simulink model "smo13"  (R2023a)
settings: Solver=VariableStepAuto  StartTime=0.0  StopTime=100  RelTol=1e-3
model workspace (MAT data in the model file):
  MaxTaskWeight = 2
  lambda = 1
  mu = 1
values from neighbouring files (symbols this model uses):
  m = m + 1    (= 2)    [TMO5liubimov.m]    (also in laba2.m = 14; laba3.m = 200; test.m = 5)
  n = 31    [laba2.m]    (also in test.m = 7)
settings Model: PacingRate=1000  Creator=error  LastModifiedBy=error

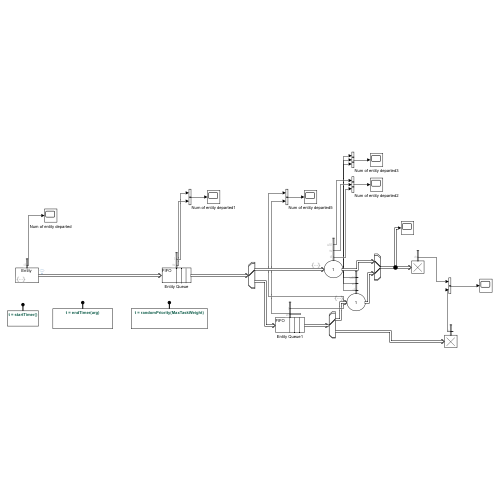
[thumbnail: Simulink's stored preview of the top-level diagram]
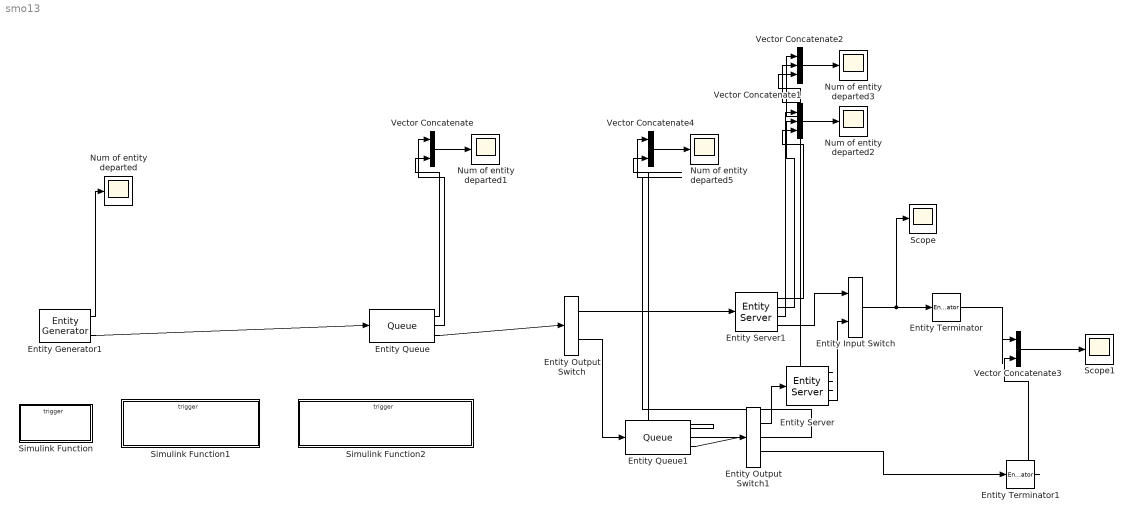
== system smo13 ==
  Entity Input Switch : EntityInputSwitch  InputPortMessageModes=m,m  OutputPortMessageModes=m
  Entity Output Switch : EntityOutputSwitch  InputPortMessageModes=m  OutputPortMessageModes=m,m  SwitchAttributeName=Attribute1
  Entity Output Switch1 : EntityOutputSwitch  InputPortMessageModes=m  OutputPortMessageModes=m,m  SwitchAttributeName=Attribute1
  Entity Generator1 : EntityGenerator  OutputPortMessageModes=n,m  TimeSource=MATLAB action  IntergenerationTimeAction=|  GenerateAction=|  AttributeName=ServiceTime|arrivalTime|time|priority  AttributeInitialValue=exprnd(1/mu);|0|0|0  NumberEntitiesDeparted=on  EntityType=Structured  EntityTypeName=Entity
      IntergenerationTimeAction=|
      | persistent rngInit;
      | if isempty(rngInit)
      |     rng(12345);
      |     rngInit = true;
      | end
      | 
      | dt = exprnd(1/lambda);
      GenerateAction=|
      | entity.arrivalTime = startTimer();
      | entity.priority = randomPriority(MaxTaskWeight+5);
      settings: OutputPortMap=o0,o3
  Entity Queue : Queue  InputPortMessageModes=m  OutputPortMessageModes=n,n,m  AverageWait=on  AverageQueueLength=on
      settings: OutputPortMap=o2,o3,o5
  Entity Queue1 : Queue  InputPortMessageModes=m  OutputPortMessageModes=n,n,m  Capacity=1  PrioritySource=priority  AverageWait=on  AverageQueueLength=on
      settings: OutputPortMap=o2,o3,o5
  Entity Server : EntityServer  InputPortMessageModes=m  OutputPortMessageModes=n,n,n,m  Capacity=1  ServiceTimeSource=Attribute  EntryAction=|  NumberEntitiesDeparted=on  AverageWait=on  Utilization=on
      | entity.time = endTimer(entity.arrivalTime);
      | 
      | i = rand();
      | 
      | if i < 0.8
      |     fprintf("Pause 2\n");
      |     pause(5);
      | end
      settings: OutputPortMap=o0,o4,o5,o9
  Entity Server1 : EntityServer  InputPortMessageModes=m  OutputPortMessageModes=n,n,n,m  Capacity=1  ServiceTimeSource=Attribute  EntryAction=|  NumberEntitiesDeparted=on  AverageWait=on  Utilization=on
      | entity.time = endTimer(entity.arrivalTime);
      | 
      | i = rand();
      | 
      | if i < 0.8
      |     fprintf("Pause 1\n");
      |     pause(5);
      | end
      settings: OutputPortMap=o0,o4,o5,o9
  Entity Terminator : EntityTerminator  InputPortMessageModes=m  NumberEntitiesArrived=on
      settings: OutputPortMap=o0
  Entity Terminator1 : EntityTerminator  InputPortMessageModes=m  NumberEntitiesArrived=on
      settings: OutputPortMap=o0
  Num of entity departed{,1..3,5} (5 alike) : Scope
  Scope : Scope
  Scope1 : Scope
  Simulink Function : Subsystem  TreatAsAtomicUnit=on
  Simulink Function1 : Subsystem  TreatAsAtomicUnit=on
  Simulink Function2 : Subsystem  TreatAsAtomicUnit=on
  Vector Concatenate : Concatenate
  Vector Concatenate1 : Concatenate  NumInputs=3
  Vector Concatenate2 : Concatenate  NumInputs=3
  Vector Concatenate3 : Concatenate
  Vector Concatenate4 : Concatenate
  wires:
  Entity Generator1/1 -> Num of entity departed/1
  Entity Generator1/2 -> Entity Queue/1
  Entity Queue/3 -> Entity Output Switch/1
  Entity Output Switch/1 -> Entity Server1/1
  Entity Output Switch/2 -> Entity Queue1/1
  Entity Server1/4 -> Entity Input Switch/1
  Entity Queue1/3 -> Entity Output Switch1/1
  Entity Output Switch1/1 -> Entity Server/1
  Entity Server/4 -> Entity Input Switch/2
  Entity Output Switch1/2 -> Entity Terminator1/1
  Entity Input Switch/1 -> Scope/1, Entity Terminator/1
  Vector Concatenate/1 -> Num of entity departed1/1
  Entity Queue/2 -> Vector Concatenate/1
  Entity Queue/1 -> Vector Concatenate/2
  Vector Concatenate1/1 -> Num of entity departed2/1
  Entity Server1/3 -> Vector Concatenate1/1
  Entity Server1/2 -> Vector Concatenate1/2
  Entity Server1/1 -> Vector Concatenate1/3
  Vector Concatenate2/1 -> Num of entity departed3/1
  Entity Server/3 -> Vector Concatenate2/1
  Entity Server/2 -> Vector Concatenate2/2
  Entity Server/1 -> Vector Concatenate2/3
  Entity Terminator/1 -> Vector Concatenate3/1
  Entity Terminator1/1 -> Vector Concatenate3/2
  Vector Concatenate3/1 -> Scope1/1
  Vector Concatenate4/1 -> Num of entity departed5/1
  Entity Queue1/2 -> Vector Concatenate4/1
  Entity Queue1/1 -> Vector Concatenate4/2

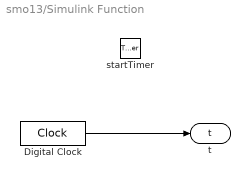
== system smo13/Simulink Function ==
  startTimer : TriggerPort  TriggerType=function-call  IsSimulinkFunction=on  FunctionName=startTimer  FunctionVisibility=scoped  VariantControl=(inherit)
  Digital Clock : DigitalClock  SampleTime=-1
  t : ArgOut  DisableCoverage=on  ArgumentName=t
  wires:
  Digital Clock/1 -> t/1

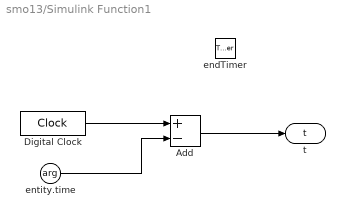
== system smo13/Simulink Function1 ==
  endTimer : TriggerPort  TriggerType=function-call  IsSimulinkFunction=on  FunctionName=endTimer  FunctionVisibility=scoped  VariantControl=(inherit)
  Add : Sum  Inputs=+-
  Digital Clock : DigitalClock  SampleTime=-1
  entity.time : ArgIn  ArgumentName=arg
  t : ArgOut  DisableCoverage=on  ArgumentName=t
  wires:
  Digital Clock/1 -> Add/1
  entity.time/1 -> Add/2
  Add/1 -> t/1

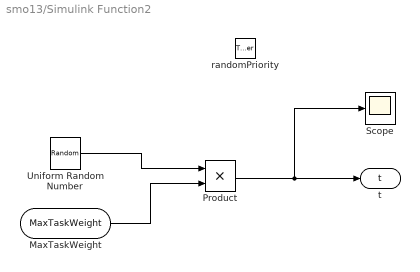
== system smo13/Simulink Function2 ==
  randomPriority : TriggerPort  TriggerType=function-call  IsSimulinkFunction=on  FunctionName=randomPriority  FunctionVisibility=scoped  VariantControl=(inherit)
  Product : Product
  Scope : Scope
  Uniform Random Number : UniformRandomNumber  Minimum=0  Seed=12345  VectorParams1D=off
  MaxTaskWeight : ArgIn  ArgumentName=MaxTaskWeight
  t : ArgOut  DisableCoverage=on  ArgumentName=t
  wires:
  Uniform Random Number/1 -> Product/1
  MaxTaskWeight/1 -> Product/2
  Product/1 -> Scope/1, t/1
